simulink library "halout"  (R2021b)
settings: Solver=VariableStepAuto  StartTime=0.0  StopTime=10.0  RelTol=1e-3
undefined symbols (not defined in the file): C_TASK_5MS_S, FALSE, KHAL_CAN1FDAPS3E2E_flg, KHAL_CAN1FDAPS3TxReq_flg, KHAL_CAN1FDVCU2E2E_flg, KHAL_CAN1FDVCU2TxReq_flg, KHAL_CAN1FDVCU3E2E_flg, KHAL_CAN1FDVCU3TxReq_flg, KHAL_CAN1TxReq_flg, KHAL_CAN2TxReq_flg, KHAL_CAN3FDVCU1TxReq_flg, KHAL_CAN3FDVCU2E2E_flg, KHAL_CAN3FDVCU2TxReq_flg, KHAL_CAN3TxReq_flg, KHAL_CAN4FDVCU1E2E_flg, KHAL_CAN4FDVCU1TxReq_flg, KHAL_CAN4TxReq_flg, KHAL_CAN5TxReq_flg, ONE_INT, TRUE, ZERO_INT
libraries: FVT_lib x383, simulink x179
(part 13 of 20)

== system halout/HAL_OUT/CAN1/FD_VCU3_0x159/Byte_19 ==
  Fr_EDURealDrvOrBRgnTq : Inport
  BitwiseOR : simulink/Logic and Bit Operations/Bitwise Operator  logicop=OR  UseBitMask=off  BitMask=bin2dec('11011001')  BitMaskRealWorld=Stored Integer
  SignalPack : FVT_lib/hal/SignalPack  RightShiftCnt=0  BitMask=2^8-1  LeftShiftCnt=0
  UnitConverter : DataTypeConversion  OutDataTypeStr=uint8  RndMeth=Round
  UnitConverter1 : DataTypeConversion  OutDataTypeStr=uint16  RndMeth=Round
  convert_out : FVT_lib/hal/convert_out  gain=0.5  offset=-5300
  Byte_19 : Outport
  wires:
  BitwiseOR/1 -> Byte_19/1
  UnitConverter/1 -> BitwiseOR/1
  SignalPack/1 -> UnitConverter/1
  UnitConverter1/1 -> SignalPack/1
  convert_out/1 -> UnitConverter1/1
  Fr_EDURealDrvOrBRgnTq/1 -> convert_out/1

== system halout/HAL_OUT/CAN1/FD_VCU3_0x159/Byte_3 ==
  Fr_EDUSpdValid : Inport
  Fr_RgnDecrSta : Inport  Port=2
  Fr_RgnPermSta : Inport  Port=3
  RgnAbnorSta : Inport  Port=4
  Rr_EDUSpdValid : Inport  Port=5
  Rr_RgnDecrSta : Inport  Port=6
  Rr_RgnPermSta : Inport  Port=7
  BitwiseOR : simulink/Logic and Bit Operations/Bitwise Operator  logicop=OR  UseBitMask=off  NumInputPorts=7  BitMask=bin2dec('11011001')  BitMaskRealWorld=Stored Integer
  SignalPack : FVT_lib/hal/SignalPack  RightShiftCnt=0  BitMask=2^1-1  LeftShiftCnt=6
  SignalPack1 : FVT_lib/hal/SignalPack  RightShiftCnt=0  BitMask=2^1-1  LeftShiftCnt=3
  SignalPack2 : FVT_lib/hal/SignalPack  RightShiftCnt=0  BitMask=2^1-1  LeftShiftCnt=1
  SignalPack3 : FVT_lib/hal/SignalPack  RightShiftCnt=0  BitMask=2^1-1  LeftShiftCnt=4
  SignalPack4 : FVT_lib/hal/SignalPack  RightShiftCnt=0  BitMask=2^1-1  LeftShiftCnt=5
  SignalPack5 : FVT_lib/hal/SignalPack  RightShiftCnt=0  BitMask=2^1-1  LeftShiftCnt=2
  SignalPack6 : FVT_lib/hal/SignalPack  RightShiftCnt=0  BitMask=2^1-1  LeftShiftCnt=0
  UnitConverter{,1..13} (14 alike) : DataTypeConversion  OutDataTypeStr=uint8  RndMeth=Round
  Byte_3 : Outport
  wires:
  BitwiseOR/1 -> Byte_3/1
  UnitConverter/1 -> BitwiseOR/1
  SignalPack/1 -> UnitConverter/1
  UnitConverter1/1 -> SignalPack/1
  Fr_EDUSpdValid/1 -> UnitConverter1/1
  UnitConverter2/1 -> BitwiseOR/2
  SignalPack1/1 -> UnitConverter2/1
  UnitConverter3/1 -> SignalPack1/1
  Fr_RgnDecrSta/1 -> UnitConverter3/1
  UnitConverter4/1 -> BitwiseOR/3
  SignalPack2/1 -> UnitConverter4/1
  UnitConverter5/1 -> SignalPack2/1
  Fr_RgnPermSta/1 -> UnitConverter5/1
  UnitConverter6/1 -> BitwiseOR/4
  SignalPack3/1 -> UnitConverter6/1
  UnitConverter7/1 -> SignalPack3/1
  RgnAbnorSta/1 -> UnitConverter7/1
  UnitConverter8/1 -> BitwiseOR/5
  SignalPack4/1 -> UnitConverter8/1
  UnitConverter9/1 -> SignalPack4/1
  Rr_EDUSpdValid/1 -> UnitConverter9/1
  UnitConverter10/1 -> BitwiseOR/6
  SignalPack5/1 -> UnitConverter10/1
  UnitConverter11/1 -> SignalPack5/1
  Rr_RgnDecrSta/1 -> UnitConverter11/1
  UnitConverter12/1 -> BitwiseOR/7
  SignalPack6/1 -> UnitConverter12/1
  UnitConverter13/1 -> SignalPack6/1
  Rr_RgnPermSta/1 -> UnitConverter13/1

== system halout/HAL_OUT/CAN1/FD_VCU3_0x159/Byte_4 ==
  EquivAccPedalSWSta : Inport
  PTCS_PermSta : Inport  Port=2
  Rr_EDUSpd : Inport  Port=3
  BitwiseOR : simulink/Logic and Bit Operations/Bitwise Operator  logicop=OR  UseBitMask=off  NumInputPorts=3  BitMask=bin2dec('11011001')  BitMaskRealWorld=Stored Integer
  SignalPack : FVT_lib/hal/SignalPack  RightShiftCnt=0  BitMask=2^1-1  LeftShiftCnt=6
  SignalPack1 : FVT_lib/hal/SignalPack  RightShiftCnt=0  BitMask=2^1-1  LeftShiftCnt=7
  SignalPack2 : FVT_lib/hal/SignalPack  RightShiftCnt=8  BitMask=2^4-1  LeftShiftCnt=0
  UnitConverter{,1..4} (5 alike) : DataTypeConversion  OutDataTypeStr=uint8  RndMeth=Round
  UnitConverter5 : DataTypeConversion  OutDataTypeStr=uint16  RndMeth=Round
  convert_out : FVT_lib/hal/convert_out  gain=1  offset=-2000
  Byte_4 : Outport
  wires:
  BitwiseOR/1 -> Byte_4/1
  UnitConverter/1 -> BitwiseOR/1
  SignalPack/1 -> UnitConverter/1
  UnitConverter1/1 -> SignalPack/1
  EquivAccPedalSWSta/1 -> UnitConverter1/1
  UnitConverter2/1 -> BitwiseOR/2
  SignalPack1/1 -> UnitConverter2/1
  UnitConverter3/1 -> SignalPack1/1
  PTCS_PermSta/1 -> UnitConverter3/1
  UnitConverter4/1 -> BitwiseOR/3
  SignalPack2/1 -> UnitConverter4/1
  UnitConverter5/1 -> SignalPack2/1
  convert_out/1 -> UnitConverter5/1
  Rr_EDUSpd/1 -> convert_out/1

== system halout/HAL_OUT/CAN1/FD_VCU3_0x159/Byte_5 ==
  Rr_EDUSpd : Inport
  BitwiseOR : simulink/Logic and Bit Operations/Bitwise Operator  logicop=OR  UseBitMask=off  BitMask=bin2dec('11011001')  BitMaskRealWorld=Stored Integer
  SignalPack : FVT_lib/hal/SignalPack  RightShiftCnt=0  BitMask=2^8-1  LeftShiftCnt=0
  UnitConverter : DataTypeConversion  OutDataTypeStr=uint8  RndMeth=Round
  UnitConverter1 : DataTypeConversion  OutDataTypeStr=uint16  RndMeth=Round
  convert_out : FVT_lib/hal/convert_out  gain=1  offset=-2000
  Byte_5 : Outport
  wires:
  BitwiseOR/1 -> Byte_5/1
  UnitConverter/1 -> BitwiseOR/1
  SignalPack/1 -> UnitConverter/1
  UnitConverter1/1 -> SignalPack/1
  convert_out/1 -> UnitConverter1/1
  Rr_EDUSpd/1 -> convert_out/1

== system halout/HAL_OUT/CAN1/FD_VCU3_0x159/Byte_6 ==
  Rr_EDURealARgnTq : Inport
  BitwiseOR : simulink/Logic and Bit Operations/Bitwise Operator  logicop=OR  UseBitMask=off  BitMask=bin2dec('11011001')  BitMaskRealWorld=Stored Integer
  SignalPack : FVT_lib/hal/SignalPack  RightShiftCnt=8  BitMask=2^8-1  LeftShiftCnt=0
  UnitConverter : DataTypeConversion  OutDataTypeStr=uint8  RndMeth=Round
  UnitConverter1 : DataTypeConversion  OutDataTypeStr=uint16  RndMeth=Round
  convert_out : FVT_lib/hal/convert_out  gain=1  offset=-5300
  Byte_6 : Outport
  wires:
  BitwiseOR/1 -> Byte_6/1
  UnitConverter/1 -> BitwiseOR/1
  SignalPack/1 -> UnitConverter/1
  UnitConverter1/1 -> SignalPack/1
  convert_out/1 -> UnitConverter1/1
  Rr_EDURealARgnTq/1 -> convert_out/1

== system halout/HAL_OUT/CAN1/FD_VCU3_0x159/Byte_7 ==
  Rr_EDURealARgnTq : Inport
  BitwiseOR : simulink/Logic and Bit Operations/Bitwise Operator  logicop=OR  UseBitMask=off  BitMask=bin2dec('11011001')  BitMaskRealWorld=Stored Integer
  SignalPack : FVT_lib/hal/SignalPack  RightShiftCnt=0  BitMask=2^8-1  LeftShiftCnt=0
  UnitConverter : DataTypeConversion  OutDataTypeStr=uint8  RndMeth=Round
  UnitConverter1 : DataTypeConversion  OutDataTypeStr=uint16  RndMeth=Round
  convert_out : FVT_lib/hal/convert_out  gain=1  offset=-5300
  Byte_7 : Outport
  wires:
  BitwiseOR/1 -> Byte_7/1
  UnitConverter/1 -> BitwiseOR/1
  SignalPack/1 -> UnitConverter/1
  UnitConverter1/1 -> SignalPack/1
  convert_out/1 -> UnitConverter1/1
  Rr_EDURealARgnTq/1 -> convert_out/1

== system halout/HAL_OUT/CAN1/FD_VCU3_0x159/Byte_8 ==
  Rr_EDUAvailBrkRgnTq : Inport
  BitwiseOR : simulink/Logic and Bit Operations/Bitwise Operator  logicop=OR  UseBitMask=off  BitMask=bin2dec('11011001')  BitMaskRealWorld=Stored Integer
  SignalPack : FVT_lib/hal/SignalPack  RightShiftCnt=8  BitMask=2^8-1  LeftShiftCnt=0
  UnitConverter : DataTypeConversion  OutDataTypeStr=uint8  RndMeth=Round
  UnitConverter1 : DataTypeConversion  OutDataTypeStr=uint16  RndMeth=Round
  convert_out : FVT_lib/hal/convert_out  gain=0.5  offset=-5300
  Byte_8 : Outport
  wires:
  BitwiseOR/1 -> Byte_8/1
  UnitConverter/1 -> BitwiseOR/1
  SignalPack/1 -> UnitConverter/1
  UnitConverter1/1 -> SignalPack/1
  convert_out/1 -> UnitConverter1/1
  Rr_EDUAvailBrkRgnTq/1 -> convert_out/1

== system halout/HAL_OUT/CAN1/FD_VCU3_0x159/Byte_9 ==
  Rr_EDUAvailBrkRgnTq : Inport
  BitwiseOR : simulink/Logic and Bit Operations/Bitwise Operator  logicop=OR  UseBitMask=off  BitMask=bin2dec('11011001')  BitMaskRealWorld=Stored Integer
  SignalPack : FVT_lib/hal/SignalPack  RightShiftCnt=0  BitMask=2^8-1  LeftShiftCnt=0
  UnitConverter : DataTypeConversion  OutDataTypeStr=uint8  RndMeth=Round
  UnitConverter1 : DataTypeConversion  OutDataTypeStr=uint16  RndMeth=Round
  convert_out : FVT_lib/hal/convert_out  gain=0.5  offset=-5300
  Byte_9 : Outport
  wires:
  BitwiseOR/1 -> Byte_9/1
  UnitConverter/1 -> BitwiseOR/1
  SignalPack/1 -> UnitConverter/1
  UnitConverter1/1 -> SignalPack/1
  convert_out/1 -> UnitConverter1/1
  Rr_EDUAvailBrkRgnTq/1 -> convert_out/1

== system halout/HAL_OUT/CAN1/FD_VCU3_0x159/CSVCU3CAN1 ==
  CSVCU3CAN1 : Inport
  Data Type Conversion : DataTypeConversion  OutDataTypeStr=uint8  RndMeth=Round
  CAN1_CS_VCU3_CAN1 : Outport
  wires:
  Data Type Conversion/1 -> CAN1_CS_VCU3_CAN1/1
  CSVCU3CAN1/1 -> Data Type Conversion/1

== system halout/HAL_OUT/CAN1/FD_VCU3_0x159/EquivAccPedalSWSta ==
  EquivAccPedalSWSta : Inport
  Data Type Conversion : DataTypeConversion  OutDataTypeStr=uint8  RndMeth=Round
  CAN1_EquivAccPedalSWSta : Outport
  wires:
  Data Type Conversion/1 -> CAN1_EquivAccPedalSWSta/1
  EquivAccPedalSWSta/1 -> Data Type Conversion/1

== system halout/HAL_OUT/CAN1/FD_VCU3_0x159/FrEDUAvailBrkRgnTq ==
  FrEDUAvailBrkRgnTq : Inport
  Data Type Conversion : DataTypeConversion  OutDataTypeStr=uint16  RndMeth=Round
  convert_out : FVT_lib/hal/convert_out  gain=0.5  offset=-5300
  CAN1_Fr_EDUAvailBrkRgnTq : Outport
  wires:
  Data Type Conversion/1 -> CAN1_Fr_EDUAvailBrkRgnTq/1
  convert_out/1 -> Data Type Conversion/1
  FrEDUAvailBrkRgnTq/1 -> convert_out/1

== system halout/HAL_OUT/CAN1/FD_VCU3_0x159/FrEDUAvailBrkRgnTqValid ==
  FrEDUAvailBrkRgnTqValid : Inport
  Data Type Conversion : DataTypeConversion  OutDataTypeStr=uint8  RndMeth=Round
  CAN1_Fr_EDUAvailBrkRgnTqValid : Outport
  wires:
  Data Type Conversion/1 -> CAN1_Fr_EDUAvailBrkRgnTqValid/1
  FrEDUAvailBrkRgnTqValid/1 -> Data Type Conversion/1

== system halout/HAL_OUT/CAN1/FD_VCU3_0x159/FrEDURealARgnTq ==
  FrEDURealARgnTq : Inport
  Data Type Conversion : DataTypeConversion  OutDataTypeStr=uint16  RndMeth=Round
  convert_out : FVT_lib/hal/convert_out  gain=1  offset=-5300
  CAN1_Fr_EDURealARgnTq : Outport
  wires:
  Data Type Conversion/1 -> CAN1_Fr_EDURealARgnTq/1
  convert_out/1 -> Data Type Conversion/1
  FrEDURealARgnTq/1 -> convert_out/1

== system halout/HAL_OUT/CAN1/FD_VCU3_0x159/FrEDURealDrvOrBRgnTq ==
  FrEDURealDrvOrBRgnTq : Inport
  Data Type Conversion : DataTypeConversion  OutDataTypeStr=uint16  RndMeth=Round
  convert_out : FVT_lib/hal/convert_out  gain=0.5  offset=-5300
  CAN1_Fr_EDURealDrvOrBRgnTq : Outport
  wires:
  Data Type Conversion/1 -> CAN1_Fr_EDURealDrvOrBRgnTq/1
  convert_out/1 -> Data Type Conversion/1
  FrEDURealDrvOrBRgnTq/1 -> convert_out/1

== system halout/HAL_OUT/CAN1/FD_VCU3_0x159/FrEDUSpd ==
  FrEDUSpd : Inport
  Data Type Conversion : DataTypeConversion  OutDataTypeStr=uint16  RndMeth=Round
  convert_out : FVT_lib/hal/convert_out  gain=1  offset=-2000
  CAN1_Fr_EDUSpd : Outport
  wires:
  Data Type Conversion/1 -> CAN1_Fr_EDUSpd/1
  convert_out/1 -> Data Type Conversion/1
  FrEDUSpd/1 -> convert_out/1

== system halout/HAL_OUT/CAN1/FD_VCU3_0x159/FrEDUSpdValid ==
  FrEDUSpdValid : Inport
  Data Type Conversion : DataTypeConversion  OutDataTypeStr=uint8  RndMeth=Round
  CAN1_Fr_EDUSpdValid : Outport
  wires:
  Data Type Conversion/1 -> CAN1_Fr_EDUSpdValid/1
  FrEDUSpdValid/1 -> Data Type Conversion/1

== system halout/HAL_OUT/CAN1/FD_VCU3_0x159/FrRgnDecrSta ==
  FrRgnDecrSta : Inport
  Data Type Conversion : DataTypeConversion  OutDataTypeStr=uint8  RndMeth=Round
  CAN1_Fr_RgnDecrSta : Outport
  wires:
  Data Type Conversion/1 -> CAN1_Fr_RgnDecrSta/1
  FrRgnDecrSta/1 -> Data Type Conversion/1

== system halout/HAL_OUT/CAN1/FD_VCU3_0x159/FrRgnPermSta ==
  FrRgnPermSta : Inport
  Data Type Conversion : DataTypeConversion  OutDataTypeStr=uint8  RndMeth=Round
  CAN1_Fr_RgnPermSta : Outport
  wires:
  Data Type Conversion/1 -> CAN1_Fr_RgnPermSta/1
  FrRgnPermSta/1 -> Data Type Conversion/1

== system halout/HAL_OUT/CAN1/FD_VCU3_0x159/PTCSPermSta ==
  PTCSPermSta : Inport
  Data Type Conversion : DataTypeConversion  OutDataTypeStr=uint8  RndMeth=Round
  CAN1_PTCS_PermSta : Outport
  wires:
  Data Type Conversion/1 -> CAN1_PTCS_PermSta/1
  PTCSPermSta/1 -> Data Type Conversion/1

== system halout/HAL_OUT/CAN1/FD_VCU3_0x159/RCVCU3CAN1 ==
  RCVCU3CAN1 : Inport
  Data Type Conversion : DataTypeConversion  OutDataTypeStr=uint8  RndMeth=Round
  CAN1_RC_VCU3_CAN1 : Outport
  wires:
  Data Type Conversion/1 -> CAN1_RC_VCU3_CAN1/1
  RCVCU3CAN1/1 -> Data Type Conversion/1

== system halout/HAL_OUT/CAN1/FD_VCU3_0x159/RgnAbnorSta ==
  RgnAbnorSta : Inport
  Data Type Conversion : DataTypeConversion  OutDataTypeStr=uint8  RndMeth=Round
  CAN1_RgnAbnorSta : Outport
  wires:
  Data Type Conversion/1 -> CAN1_RgnAbnorSta/1
  RgnAbnorSta/1 -> Data Type Conversion/1

== system halout/HAL_OUT/CAN1/FD_VCU3_0x159/RrEDUAvailBrkRgnTq ==
  RrEDUAvailBrkRgnTq : Inport
  Data Type Conversion : DataTypeConversion  OutDataTypeStr=uint16  RndMeth=Round
  convert_out : FVT_lib/hal/convert_out  gain=0.5  offset=-5300
  CAN1_Rr_EDUAvailBrkRgnTq : Outport
  wires:
  Data Type Conversion/1 -> CAN1_Rr_EDUAvailBrkRgnTq/1
  convert_out/1 -> Data Type Conversion/1
  RrEDUAvailBrkRgnTq/1 -> convert_out/1

== system halout/HAL_OUT/CAN1/FD_VCU3_0x159/RrEDUAvailBrkRgnTqValid ==
  RrEDUAvailBrkRgnTqValid : Inport
  Data Type Conversion : DataTypeConversion  OutDataTypeStr=uint8  RndMeth=Round
  CAN1_Rr_EDUAvailBrkRgnTqValid : Outport
  wires:
  Data Type Conversion/1 -> CAN1_Rr_EDUAvailBrkRgnTqValid/1
  RrEDUAvailBrkRgnTqValid/1 -> Data Type Conversion/1

== system halout/HAL_OUT/CAN1/FD_VCU3_0x159/RrEDURealARgnTq ==
  RrEDURealARgnTq : Inport
  Data Type Conversion : DataTypeConversion  OutDataTypeStr=uint16  RndMeth=Round
  convert_out : FVT_lib/hal/convert_out  gain=1  offset=-5300
  CAN1_Rr_EDURealARgnTq : Outport
  wires:
  Data Type Conversion/1 -> CAN1_Rr_EDURealARgnTq/1
  convert_out/1 -> Data Type Conversion/1
  RrEDURealARgnTq/1 -> convert_out/1

== system halout/HAL_OUT/CAN1/FD_VCU3_0x159/RrEDURealDrvOrBRgnTq ==
  RrEDURealDrvOrBRgnTq : Inport
  Data Type Conversion : DataTypeConversion  OutDataTypeStr=uint16  RndMeth=Round
  convert_out : FVT_lib/hal/convert_out  gain=0.5  offset=-5300
  CAN1_Rr_EDURealDrvOrBRgnTq : Outport
  wires:
  Data Type Conversion/1 -> CAN1_Rr_EDURealDrvOrBRgnTq/1
  convert_out/1 -> Data Type Conversion/1
  RrEDURealDrvOrBRgnTq/1 -> convert_out/1

== system halout/HAL_OUT/CAN1/FD_VCU3_0x159/RrEDUSpd ==
  RrEDUSpd : Inport
  Data Type Conversion : DataTypeConversion  OutDataTypeStr=uint16  RndMeth=Round
  convert_out : FVT_lib/hal/convert_out  gain=1  offset=-2000
  CAN1_Rr_EDUSpd : Outport
  wires:
  Data Type Conversion/1 -> CAN1_Rr_EDUSpd/1
  convert_out/1 -> Data Type Conversion/1
  RrEDUSpd/1 -> convert_out/1

== system halout/HAL_OUT/CAN1/FD_VCU3_0x159/RrEDUSpdValid ==
  RrEDUSpdValid : Inport
  Data Type Conversion : DataTypeConversion  OutDataTypeStr=uint8  RndMeth=Round
  CAN1_Rr_EDUSpdValid : Outport
  wires:
  Data Type Conversion/1 -> CAN1_Rr_EDUSpdValid/1
  RrEDUSpdValid/1 -> Data Type Conversion/1

== system halout/HAL_OUT/CAN1/FD_VCU3_0x159/RrRgnDecrSta ==
  RrRgnDecrSta : Inport
  Data Type Conversion : DataTypeConversion  OutDataTypeStr=uint8  RndMeth=Round
  CAN1_Rr_RgnDecrSta : Outport
  wires:
  Data Type Conversion/1 -> CAN1_Rr_RgnDecrSta/1
  RrRgnDecrSta/1 -> Data Type Conversion/1

== system halout/HAL_OUT/CAN1/FD_VCU3_0x159/RrRgnPermSta ==
  RrRgnPermSta : Inport
  Data Type Conversion : DataTypeConversion  OutDataTypeStr=uint8  RndMeth=Round
  CAN1_Rr_RgnPermSta : Outport
  wires:
  Data Type Conversion/1 -> CAN1_Rr_RgnPermSta/1
  RrRgnPermSta/1 -> Data Type Conversion/1

== system halout/HAL_OUT/CAN1/FD_VCU4_0x3C0/EngAGSCloseSta ==
  EngAGSCloseSta : Inport
  Data Type Conversion : DataTypeConversion  OutDataTypeStr=uint8  RndMeth=Round
  CAN1_Eng_AGSCloseSta : Outport
  wires:
  Data Type Conversion/1 -> CAN1_Eng_AGSCloseSta/1
  EngAGSCloseSta/1 -> Data Type Conversion/1

== system halout/HAL_OUT/CAN1/FD_VCU4_0x3C0/EngActvDmpDisabSta ==
  EngActvDmpDisabSta : Inport
  Data Type Conversion : DataTypeConversion  OutDataTypeStr=uint8  RndMeth=Round
  CAN1_Eng_ActvDmpDisabSta : Outport
  wires:
  Data Type Conversion/1 -> CAN1_Eng_ActvDmpDisabSta/1
  EngActvDmpDisabSta/1 -> Data Type Conversion/1

== system halout/HAL_OUT/CAN1/FD_VCU4_0x3C0/EngCoastDwSta ==
  EngCoastDwSta : Inport
  Data Type Conversion : DataTypeConversion  OutDataTypeStr=uint8  RndMeth=Round
  CAN1_Eng_CoastDwSta : Outport
  wires:
  Data Type Conversion/1 -> CAN1_Eng_CoastDwSta/1
  EngCoastDwSta/1 -> Data Type Conversion/1

== system halout/HAL_OUT/CAN1/FD_VCU4_0x3C0/EngPwrLockSta ==
  EngPwrLockSta : Inport
  Data Type Conversion : DataTypeConversion  OutDataTypeStr=uint8  RndMeth=Round
  CAN1_Eng_PwrLockSta : Outport
  wires:
  Data Type Conversion/1 -> CAN1_Eng_PwrLockSta/1
  EngPwrLockSta/1 -> Data Type Conversion/1

== system halout/HAL_OUT/CAN1/FD_VCU4_0x3C0/VehMalfunLevel ==
  VehMalfunLevel : Inport
  Data Type Conversion : DataTypeConversion  OutDataTypeStr=uint8  RndMeth=Round
  CAN1_VehMalfunLevel : Outport
  wires:
  Data Type Conversion/1 -> CAN1_VehMalfunLevel/1
  VehMalfunLevel/1 -> Data Type Conversion/1

== system halout/HAL_OUT/CAN2/FD_APS1_0x236/APSAngleTarget ==
  APSAngleTarget : Inport
  Data Type Conversion : DataTypeConversion  OutDataTypeStr=uint16  RndMeth=Round
  convert_out : FVT_lib/hal/convert_out  gain=0.1  offset=-900
  CAN2_APS_Angle_Target : Outport
  wires:
  Data Type Conversion/1 -> CAN2_APS_Angle_Target/1
  convert_out/1 -> Data Type Conversion/1
  APSAngleTarget/1 -> convert_out/1

== system halout/HAL_OUT/CAN2/FD_APS1_0x236/APSRqEPASCtrl ==
  APSRqEPASCtrl : Inport
  Data Type Conversion : DataTypeConversion  OutDataTypeStr=uint8  RndMeth=Round
  CAN2_APS_Rq_EPAS_Ctrl : Outport
  wires:
  Data Type Conversion/1 -> CAN2_APS_Rq_EPAS_Ctrl/1
  APSRqEPASCtrl/1 -> Data Type Conversion/1

== system halout/HAL_OUT/CAN2/FD_APS1_0x236/APSStaSystem ==
  APSStaSystem : Inport
  Data Type Conversion : DataTypeConversion  OutDataTypeStr=uint8  RndMeth=Round
  CAN2_APS_Sta_System : Outport
  wires:
  Data Type Conversion/1 -> CAN2_APS_Sta_System/1
  APSStaSystem/1 -> Data Type Conversion/1

== system halout/HAL_OUT/CAN2/FD_APS1_0x236/APSVRqEPASCtrl ==
  APSVRqEPASCtrl : Inport
  Data Type Conversion : DataTypeConversion  OutDataTypeStr=uint8  RndMeth=Round
  CAN2_APS_V_Rq_EPAS_Ctrl : Outport
  wires:
  Data Type Conversion/1 -> CAN2_APS_V_Rq_EPAS_Ctrl/1
  APSVRqEPASCtrl/1 -> Data Type Conversion/1

== system halout/HAL_OUT/CAN2/FD_APS2_0x210/APSDFLL ==
  APSDFLL : Inport
  Data Type Conversion : DataTypeConversion  OutDataTypeStr=uint16  RndMeth=Round
  CAN2_APS_D_FLL : Outport
  wires:
  Data Type Conversion/1 -> CAN2_APS_D_FLL/1
  APSDFLL/1 -> Data Type Conversion/1

== system halout/HAL_OUT/CAN2/FD_APS2_0x210/APSDFLR ==
  APSDFLR : Inport
  Data Type Conversion : DataTypeConversion  OutDataTypeStr=uint16  RndMeth=Round
  CAN2_APS_D_FLR : Outport
  wires:
  Data Type Conversion/1 -> CAN2_APS_D_FLR/1
  APSDFLR/1 -> Data Type Conversion/1

== system halout/HAL_OUT/CAN2/FD_APS2_0x210/APSDRLL ==
  APSDRLL : Inport
  Data Type Conversion : DataTypeConversion  OutDataTypeStr=uint16  RndMeth=Round
  CAN2_APS_D_RLL : Outport
  wires:
  Data Type Conversion/1 -> CAN2_APS_D_RLL/1
  APSDRLL/1 -> Data Type Conversion/1

== system halout/HAL_OUT/CAN2/FD_APS2_0x210/APSDRLR ==
  APSDRLR : Inport
  Data Type Conversion : DataTypeConversion  OutDataTypeStr=uint16  RndMeth=Round
  CAN2_APS_D_RLR : Outport
  wires:
  Data Type Conversion/1 -> CAN2_APS_D_RLR/1
  APSDRLR/1 -> Data Type Conversion/1

== system halout/HAL_OUT/CAN2/FD_APS2_0x210/APSExitCondition ==
  APSExitCondition : Inport
  Data Type Conversion : DataTypeConversion  OutDataTypeStr=uint8  RndMeth=Round
  CAN2_APS_ExitCondition : Outport
  wires:
  Data Type Conversion/1 -> CAN2_APS_ExitCondition/1
  APSExitCondition/1 -> Data Type Conversion/1

== system halout/HAL_OUT/CAN2/FD_APS2_0x210/APSHWVer ==
  APSHWVer : Inport
  Data Type Conversion : DataTypeConversion  OutDataTypeStr=uint8  RndMeth=Round
  CAN2_APS_HW_Ver : Outport
  wires:
  Data Type Conversion/1 -> CAN2_APS_HW_Ver/1
  APSHWVer/1 -> Data Type Conversion/1

== system halout/HAL_OUT/CAN2/FD_APS2_0x210/APSProgressPCT ==
  APSProgressPCT : Inport
  Data Type Conversion : DataTypeConversion  OutDataTypeStr=uint8  RndMeth=Round
  CAN2_APS_Progress_PCT : Outport
  wires:
  Data Type Conversion/1 -> CAN2_APS_Progress_PCT/1
  APSProgressPCT/1 -> Data Type Conversion/1

== system halout/HAL_OUT/CAN2/FD_APS2_0x210/APSRQDisplay ==
  APSRQDisplay : Inport
  Data Type Conversion : DataTypeConversion  OutDataTypeStr=uint8  RndMeth=Round
  CAN2_APS_RQ_Display : Outport
  wires:
  Data Type Conversion/1 -> CAN2_APS_RQ_Display/1
  APSRQDisplay/1 -> Data Type Conversion/1

== system halout/HAL_OUT/CAN2/FD_APS2_0x210/APSSWVer ==
  APSSWVer : Inport
  Data Type Conversion : DataTypeConversion  OutDataTypeStr=uint8  RndMeth=Round
  CAN2_APS_SW_Ver : Outport
  wires:
  Data Type Conversion/1 -> CAN2_APS_SW_Ver/1
  APSSWVer/1 -> Data Type Conversion/1

== system halout/HAL_OUT/CAN2/FD_APS2_0x210/FDCVCURegenLimIndSta ==
  FDCVCURegenLimIndSta : Inport
  Data Type Conversion : DataTypeConversion  OutDataTypeStr=uint8  RndMeth=Round
  CAN2_FDC_VCU_RegenLimInd_Sta : Outport
  wires:
  Data Type Conversion/1 -> CAN2_FDC_VCU_RegenLimInd_Sta/1
  FDCVCURegenLimIndSta/1 -> Data Type Conversion/1

== system halout/HAL_OUT/CAN2/FD_APS2_0x210/FDCVCUSmartEcoSpdLimSta ==
  FDCVCUSmartEcoSpdLimSta : Inport
  Data Type Conversion : DataTypeConversion  OutDataTypeStr=uint8  RndMeth=Round
  CAN2_FDC_VCU_SmartEcoSpdLim_Sta : Outport
  wires:
  Data Type Conversion/1 -> CAN2_FDC_VCU_SmartEcoSpdLim_Sta/1
  FDCVCUSmartEcoSpdLimSta/1 -> Data Type Conversion/1

== system halout/HAL_OUT/CAN2/FD_APS2_0x210/FDCVCUSmartEcoSta ==
  FDCVCUSmartEcoSta : Inport
  Data Type Conversion : DataTypeConversion  OutDataTypeStr=uint8  RndMeth=Round
  CAN2_FDC_VCU_SmartEco_Sta : Outport
  wires:
  Data Type Conversion/1 -> CAN2_FDC_VCU_SmartEco_Sta/1
  FDCVCUSmartEcoSta/1 -> Data Type Conversion/1

== system halout/HAL_OUT/CAN2/FD_APS2_0x210/PASAFCL ==
  PASAFCL : Inport
  Data Type Conversion : DataTypeConversion  OutDataTypeStr=uint8  RndMeth=Round
  CAN2_PAS_A_FCL : Outport
  wires:
  Data Type Conversion/1 -> CAN2_PAS_A_FCL/1
  PASAFCL/1 -> Data Type Conversion/1

== system halout/HAL_OUT/CAN2/FD_APS2_0x210/PASAFCR ==
  PASAFCR : Inport
  Data Type Conversion : DataTypeConversion  OutDataTypeStr=uint8  RndMeth=Round
  CAN2_PAS_A_FCR : Outport
  wires:
  Data Type Conversion/1 -> CAN2_PAS_A_FCR/1
  PASAFCR/1 -> Data Type Conversion/1

== system halout/HAL_OUT/CAN2/FD_APS2_0x210/PASAFML ==
  PASAFML : Inport
  Data Type Conversion : DataTypeConversion  OutDataTypeStr=uint8  RndMeth=Round
  CAN2_PAS_A_FML : Outport
  wires:
  Data Type Conversion/1 -> CAN2_PAS_A_FML/1
  PASAFML/1 -> Data Type Conversion/1

== system halout/HAL_OUT/CAN2/FD_APS2_0x210/PASAFMR ==
  PASAFMR : Inport
  Data Type Conversion : DataTypeConversion  OutDataTypeStr=uint8  RndMeth=Round
  CAN2_PAS_A_FMR : Outport
  wires:
  Data Type Conversion/1 -> CAN2_PAS_A_FMR/1
  PASAFMR/1 -> Data Type Conversion/1

== system halout/HAL_OUT/CAN2/FD_APS2_0x210/PASARCL ==
  PASARCL : Inport
  Data Type Conversion : DataTypeConversion  OutDataTypeStr=uint8  RndMeth=Round
  CAN2_PAS_A_RCL : Outport
  wires:
  Data Type Conversion/1 -> CAN2_PAS_A_RCL/1
  PASARCL/1 -> Data Type Conversion/1

== system halout/HAL_OUT/CAN2/FD_APS2_0x210/PASARCR ==
  PASARCR : Inport
  Data Type Conversion : DataTypeConversion  OutDataTypeStr=uint8  RndMeth=Round
  CAN2_PAS_A_RCR : Outport
  wires:
  Data Type Conversion/1 -> CAN2_PAS_A_RCR/1
  PASARCR/1 -> Data Type Conversion/1

== system halout/HAL_OUT/CAN2/FD_APS2_0x210/PASARML ==
  PASARML : Inport
  Data Type Conversion : DataTypeConversion  OutDataTypeStr=uint8  RndMeth=Round
  CAN2_PAS_A_RML : Outport
  wires:
  Data Type Conversion/1 -> CAN2_PAS_A_RML/1
  PASARML/1 -> Data Type Conversion/1

== system halout/HAL_OUT/CAN2/FD_APS2_0x210/PASARMR ==
  PASARMR : Inport
  Data Type Conversion : DataTypeConversion  OutDataTypeStr=uint8  RndMeth=Round
  CAN2_PAS_A_RMR : Outport
  wires:
  Data Type Conversion/1 -> CAN2_PAS_A_RMR/1
  PASARMR/1 -> Data Type Conversion/1

== system halout/HAL_OUT/CAN2/FD_APS2_0x210/PASChime ==
  PASChime : Inport
  Data Type Conversion : DataTypeConversion  OutDataTypeStr=uint8  RndMeth=Round
  CAN2_PAS_Chime : Outport
  wires:
  Data Type Conversion/1 -> CAN2_PAS_Chime/1
  PASChime/1 -> Data Type Conversion/1

== system halout/HAL_OUT/CAN2/FD_APS2_0x210/PASDFCL ==
  PASDFCL : Inport
  Data Type Conversion : DataTypeConversion  OutDataTypeStr=uint8  RndMeth=Round
  CAN2_PAS_D_FCL : Outport
  wires:
  Data Type Conversion/1 -> CAN2_PAS_D_FCL/1
  PASDFCL/1 -> Data Type Conversion/1

== system halout/HAL_OUT/CAN2/FD_APS2_0x210/PASDFCR ==
  PASDFCR : Inport
  Data Type Conversion : DataTypeConversion  OutDataTypeStr=uint8  RndMeth=Round
  CAN2_PAS_D_FCR : Outport
  wires:
  Data Type Conversion/1 -> CAN2_PAS_D_FCR/1
  PASDFCR/1 -> Data Type Conversion/1

== system halout/HAL_OUT/CAN2/FD_APS2_0x210/PASDFML ==
  PASDFML : Inport
  Data Type Conversion : DataTypeConversion  OutDataTypeStr=uint8  RndMeth=Round
  CAN2_PAS_D_FML : Outport
  wires:
  Data Type Conversion/1 -> CAN2_PAS_D_FML/1
  PASDFML/1 -> Data Type Conversion/1

== system halout/HAL_OUT/CAN2/FD_APS2_0x210/PASDFMR ==
  PASDFMR : Inport
  Data Type Conversion : DataTypeConversion  OutDataTypeStr=uint8  RndMeth=Round
  CAN2_PAS_D_FMR : Outport
  wires:
  Data Type Conversion/1 -> CAN2_PAS_D_FMR/1
  PASDFMR/1 -> Data Type Conversion/1

== system halout/HAL_OUT/CAN2/FD_APS2_0x210/PASDRCL ==
  PASDRCL : Inport
  Data Type Conversion : DataTypeConversion  OutDataTypeStr=uint8  RndMeth=Round
  CAN2_PAS_D_RCL : Outport
  wires:
  Data Type Conversion/1 -> CAN2_PAS_D_RCL/1
  PASDRCL/1 -> Data Type Conversion/1

== system halout/HAL_OUT/CAN2/FD_APS2_0x210/PASDRCR ==
  PASDRCR : Inport
  Data Type Conversion : DataTypeConversion  OutDataTypeStr=uint8  RndMeth=Round
  CAN2_PAS_D_RCR : Outport
  wires:
  Data Type Conversion/1 -> CAN2_PAS_D_RCR/1
  PASDRCR/1 -> Data Type Conversion/1

== system halout/HAL_OUT/CAN2/FD_APS2_0x210/PASDRML ==
  PASDRML : Inport
  Data Type Conversion : DataTypeConversion  OutDataTypeStr=uint8  RndMeth=Round
  CAN2_PAS_D_RML : Outport
  wires:
  Data Type Conversion/1 -> CAN2_PAS_D_RML/1
  PASDRML/1 -> Data Type Conversion/1

== system halout/HAL_OUT/CAN2/FD_APS2_0x210/PASDRMR ==
  PASDRMR : Inport
  Data Type Conversion : DataTypeConversion  OutDataTypeStr=uint8  RndMeth=Round
  CAN2_PAS_D_RMR : Outport
  wires:
  Data Type Conversion/1 -> CAN2_PAS_D_RMR/1
  PASDRMR/1 -> Data Type Conversion/1

== system halout/HAL_OUT/CAN2/FD_APS2_0x210/PASModOperation ==
  PASModOperation : Inport
  Data Type Conversion : DataTypeConversion  OutDataTypeStr=uint8  RndMeth=Round
  CAN2_PAS_Mod_Operation : Outport
  wires:
  Data Type Conversion/1 -> CAN2_PAS_Mod_Operation/1
  PASModOperation/1 -> Data Type Conversion/1

== system halout/HAL_OUT/CAN2/FD_APS2_0x210/PASSNSRLayout ==
  PASSNSRLayout : Inport
  Data Type Conversion : DataTypeConversion  OutDataTypeStr=uint8  RndMeth=Round
  CAN2_PAS_SNSR_Layout : Outport
  wires:
  Data Type Conversion/1 -> CAN2_PAS_SNSR_Layout/1
  PASSNSRLayout/1 -> Data Type Conversion/1

== system halout/HAL_OUT/CAN2/FD_APS2_0x210/PASStaFSys ==
  PASStaFSys : Inport
  Data Type Conversion : DataTypeConversion  OutDataTypeStr=uint8  RndMeth=Round
  CAN2_PAS_Sta_F_Sys : Outport
  wires:
  Data Type Conversion/1 -> CAN2_PAS_Sta_F_Sys/1
  PASStaFSys/1 -> Data Type Conversion/1

== system halout/HAL_OUT/CAN2/FD_APS2_0x210/USSStaFCL ==
  USSStaFCL : Inport
  Data Type Conversion : DataTypeConversion  OutDataTypeStr=uint8  RndMeth=Round
  CAN2_USS_Sta_FCL : Outport
  wires:
  Data Type Conversion/1 -> CAN2_USS_Sta_FCL/1
  USSStaFCL/1 -> Data Type Conversion/1

== system halout/HAL_OUT/CAN2/FD_APS2_0x210/USSStaFCR ==
  USSStaFCR : Inport
  Data Type Conversion : DataTypeConversion  OutDataTypeStr=uint8  RndMeth=Round
  CAN2_USS_Sta_FCR : Outport
  wires:
  Data Type Conversion/1 -> CAN2_USS_Sta_FCR/1
  USSStaFCR/1 -> Data Type Conversion/1

== system halout/HAL_OUT/CAN2/FD_APS2_0x210/USSStaFLL ==
  USSStaFLL : Inport
  Data Type Conversion : DataTypeConversion  OutDataTypeStr=uint8  RndMeth=Round
  CAN2_USS_Sta_FLL : Outport
  wires:
  Data Type Conversion/1 -> CAN2_USS_Sta_FLL/1
  USSStaFLL/1 -> Data Type Conversion/1

== system halout/HAL_OUT/CAN2/FD_APS2_0x210/USSStaFLR ==
  USSStaFLR : Inport
  Data Type Conversion : DataTypeConversion  OutDataTypeStr=uint8  RndMeth=Round
  CAN2_USS_Sta_FLR : Outport
  wires:
  Data Type Conversion/1 -> CAN2_USS_Sta_FLR/1
  USSStaFLR/1 -> Data Type Conversion/1

== system halout/HAL_OUT/CAN2/FD_APS2_0x210/USSStaFML ==
  USSStaFML : Inport
  Data Type Conversion : DataTypeConversion  OutDataTypeStr=uint8  RndMeth=Round
  CAN2_USS_Sta_FML : Outport
  wires:
  Data Type Conversion/1 -> CAN2_USS_Sta_FML/1
  USSStaFML/1 -> Data Type Conversion/1

== system halout/HAL_OUT/CAN2/FD_APS2_0x210/USSStaFMR ==
  USSStaFMR : Inport
  Data Type Conversion : DataTypeConversion  OutDataTypeStr=uint8  RndMeth=Round
  CAN2_USS_Sta_FMR : Outport
  wires:
  Data Type Conversion/1 -> CAN2_USS_Sta_FMR/1
  USSStaFMR/1 -> Data Type Conversion/1

== system halout/HAL_OUT/CAN2/FD_APS2_0x210/USSStaRCL ==
  USSStaRCL : Inport
  Data Type Conversion : DataTypeConversion  OutDataTypeStr=uint8  RndMeth=Round
  CAN2_USS_Sta_RCL : Outport
  wires:
  Data Type Conversion/1 -> CAN2_USS_Sta_RCL/1
  USSStaRCL/1 -> Data Type Conversion/1

== system halout/HAL_OUT/CAN2/FD_APS2_0x210/USSStaRCR ==
  USSStaRCR : Inport
  Data Type Conversion : DataTypeConversion  OutDataTypeStr=uint8  RndMeth=Round
  CAN2_USS_Sta_RCR : Outport
  wires:
  Data Type Conversion/1 -> CAN2_USS_Sta_RCR/1
  USSStaRCR/1 -> Data Type Conversion/1

== system halout/HAL_OUT/CAN2/FD_APS2_0x210/USSStaRLL ==
  USSStaRLL : Inport
  Data Type Conversion : DataTypeConversion  OutDataTypeStr=uint8  RndMeth=Round
  CAN2_USS_Sta_RLL : Outport
  wires:
  Data Type Conversion/1 -> CAN2_USS_Sta_RLL/1
  USSStaRLL/1 -> Data Type Conversion/1

== system halout/HAL_OUT/CAN2/FD_APS2_0x210/USSStaRLR ==
  USSStaRLR : Inport
  Data Type Conversion : DataTypeConversion  OutDataTypeStr=uint8  RndMeth=Round
  CAN2_USS_Sta_RLR : Outport
  wires:
  Data Type Conversion/1 -> CAN2_USS_Sta_RLR/1
  USSStaRLR/1 -> Data Type Conversion/1

== system halout/HAL_OUT/CAN2/FD_APS2_0x210/USSStaRML ==
  USSStaRML : Inport
  Data Type Conversion : DataTypeConversion  OutDataTypeStr=uint8  RndMeth=Round
  CAN2_USS_Sta_RML : Outport
  wires:
  Data Type Conversion/1 -> CAN2_USS_Sta_RML/1
  USSStaRML/1 -> Data Type Conversion/1

== system halout/HAL_OUT/CAN2/FD_APS2_0x210/USSStaRMR ==
  USSStaRMR : Inport
  Data Type Conversion : DataTypeConversion  OutDataTypeStr=uint8  RndMeth=Round
  CAN2_USS_Sta_RMR : Outport
  wires:
  Data Type Conversion/1 -> CAN2_USS_Sta_RMR/1
  USSStaRMR/1 -> Data Type Conversion/1

== system halout/HAL_OUT/CAN2/FD_APS3_0x238/APS3LifeCount ==
  APS3LifeCount : Inport
  Data Type Conversion : DataTypeConversion  OutDataTypeStr=uint8  RndMeth=Round
  CAN2_APS3_LifeCount : Outport
  wires:
  Data Type Conversion/1 -> CAN2_APS3_LifeCount/1
  APS3LifeCount/1 -> Data Type Conversion/1

== system halout/HAL_OUT/CAN2/FD_APS3_0x238/APS3checksum ==
  APS3checksum : Inport
  Data Type Conversion : DataTypeConversion  OutDataTypeStr=uint8  RndMeth=Round
  CAN2_APS3_checksum : Outport
  wires:
  Data Type Conversion/1 -> CAN2_APS3_checksum/1
  APS3checksum/1 -> Data Type Conversion/1

== system halout/HAL_OUT/CAN2/FD_APS3_0x238/APSDecReq ==
  APSDecReq : Inport
  Data Type Conversion : DataTypeConversion  OutDataTypeStr=uint8  RndMeth=Round
  convert_out : FVT_lib/hal/convert_out  gain=0.1  offset=0
  CAN2_APS_DecReq : Outport
  wires:
  Data Type Conversion/1 -> CAN2_APS_DecReq/1
  convert_out/1 -> Data Type Conversion/1
  APSDecReq/1 -> convert_out/1

== system halout/HAL_OUT/CAN2/FD_APS3_0x238/APSDecReqA ==
  APSDecReqA : Inport
  Data Type Conversion : DataTypeConversion  OutDataTypeStr=uint8  RndMeth=Round
  CAN2_APS_DecReq_A : Outport
  wires:
  Data Type Conversion/1 -> CAN2_APS_DecReq_A/1
  APSDecReqA/1 -> Data Type Conversion/1

== system halout/HAL_OUT/CAN2/FD_APS3_0x238/APSOpenPTG ==
  APSOpenPTG : Inport
  Data Type Conversion : DataTypeConversion  OutDataTypeStr=uint8  RndMeth=Round
  CAN2_APSOpenPTG : Outport
  wires:
  Data Type Conversion/1 -> CAN2_APSOpenPTG/1
  APSOpenPTG/1 -> Data Type Conversion/1

== system halout/HAL_OUT/CAN2/FD_APS3_0x238/APSReq ==
  APSReq : Inport
  Data Type Conversion : DataTypeConversion  OutDataTypeStr=uint8  RndMeth=Round
  CAN2_APS_Req : Outport
  wires:
  Data Type Conversion/1 -> CAN2_APS_Req/1
  APSReq/1 -> Data Type Conversion/1

== system halout/HAL_OUT/CAN2/FD_APS3_0x238/CAASSta ==
  CAASSta : Inport
  Data Type Conversion : DataTypeConversion  OutDataTypeStr=uint8  RndMeth=Round
  CAN2_CAAS_Sta : Outport
  wires:
  Data Type Conversion/1 -> CAN2_CAAS_Sta/1
  CAASSta/1 -> Data Type Conversion/1

== system halout/HAL_OUT/CAN2/FD_APS3_0x238/SPTGDet ==
  SPTGDet : Inport
  Data Type Conversion : DataTypeConversion  OutDataTypeStr=uint8  RndMeth=Round
  CAN2_SPTGDet : Outport
  wires:
  Data Type Conversion/1 -> CAN2_SPTGDet/1
  SPTGDet/1 -> Data Type Conversion/1

== system halout/HAL_OUT/CAN2/FD_APS3_0x238/SPTGSta ==
  SPTGSta : Inport
  Data Type Conversion : DataTypeConversion  OutDataTypeStr=uint8  RndMeth=Round
  CAN2_SPTG_Sta : Outport
  wires:
  Data Type Conversion/1 -> CAN2_SPTG_Sta/1
  SPTGSta/1 -> Data Type Conversion/1

== system halout/HAL_OUT/CAN2/FD_BCM1_0x216/APMDoorControlSta ==
  APMDoorControlSta : Inport
  Data Type Conversion : DataTypeConversion  OutDataTypeStr=uint8  RndMeth=Round
  CAN2_APMDoorControlSta : Outport
  wires:
  Data Type Conversion/1 -> CAN2_APMDoorControlSta/1
  APMDoorControlSta/1 -> Data Type Conversion/1

== system halout/HAL_OUT/CAN2/FD_BCM1_0x216/AllDoorSW ==
  AllDoorSW : Inport
  Data Type Conversion : DataTypeConversion  OutDataTypeStr=uint8  RndMeth=Round
  CAN2_AllDoorSW : Outport
  wires:
  Data Type Conversion/1 -> CAN2_AllDoorSW/1
  AllDoorSW/1 -> Data Type Conversion/1

== system halout/HAL_OUT/CAN2/FD_BCM1_0x216/AntiTheftSeatFold ==
  AntiTheftSeatFold : Inport
  Data Type Conversion : DataTypeConversion  OutDataTypeStr=uint8  RndMeth=Round
  CAN2_AntiTheftSeatFold : Outport
  wires:
  Data Type Conversion/1 -> CAN2_AntiTheftSeatFold/1
  AntiTheftSeatFold/1 -> Data Type Conversion/1

== system halout/HAL_OUT/CAN2/FD_BCM1_0x216/AntitheftSta ==
  AntitheftSta : Inport
  Data Type Conversion : DataTypeConversion  OutDataTypeStr=uint8  RndMeth=Round
  CAN2_AntitheftSta : Outport
  wires:
  Data Type Conversion/1 -> CAN2_AntitheftSta/1
  AntitheftSta/1 -> Data Type Conversion/1

== system halout/HAL_OUT/CAN2/FD_BCM1_0x216/BCMBuzzerReq ==
  BCMBuzzerReq : Inport
  Data Type Conversion : DataTypeConversion  OutDataTypeStr=uint8  RndMeth=Round
  CAN2_BCM_Buzzer_Req : Outport
  wires:
  Data Type Conversion/1 -> CAN2_BCM_Buzzer_Req/1
  BCMBuzzerReq/1 -> Data Type Conversion/1

== system halout/HAL_OUT/CAN2/FD_BCM1_0x216/BCMDoorLockSta ==
  BCMDoorLockSta : Inport
  Data Type Conversion : DataTypeConversion  OutDataTypeStr=uint8  RndMeth=Round
  CAN2_BCM_DoorLock_Sta : Outport
  wires:
  Data Type Conversion/1 -> CAN2_BCM_DoorLock_Sta/1
  BCMDoorLockSta/1 -> Data Type Conversion/1

== system halout/HAL_OUT/CAN2/FD_BCM1_0x216/BrakeLamp ==
  BrakeLamp : Inport
  Data Type Conversion : DataTypeConversion  OutDataTypeStr=uint8  RndMeth=Round
  CAN2_BrakeLamp : Outport
  wires:
  Data Type Conversion/1 -> CAN2_BrakeLamp/1
  BrakeLamp/1 -> Data Type Conversion/1

== system halout/HAL_OUT/CAN2/FD_BCM1_0x216/CTDCtrl ==
  CTDCtrl : Inport
  Data Type Conversion : DataTypeConversion  OutDataTypeStr=uint8  RndMeth=Round
  CAN2_CTDCtrl : Outport
  wires:
  Data Type Conversion/1 -> CAN2_CTDCtrl/1
  CTDCtrl/1 -> Data Type Conversion/1

== system halout/HAL_OUT/CAN2/FD_BCM1_0x216/CTDLockSW ==
  CTDLockSW : Inport
  Data Type Conversion : DataTypeConversion  OutDataTypeStr=uint8  RndMeth=Round
  CAN2_CTDLockSW : Outport
  wires:
  Data Type Conversion/1 -> CAN2_CTDLockSW/1
  CTDLockSW/1 -> Data Type Conversion/1

== system halout/HAL_OUT/CAN2/FD_BCM1_0x216/CTDUnlockSW ==
  CTDUnlockSW : Inport
  Data Type Conversion : DataTypeConversion  OutDataTypeStr=uint8  RndMeth=Round
  CAN2_CTDUnlockSW : Outport
  wires:
  Data Type Conversion/1 -> CAN2_CTDUnlockSW/1
  CTDUnlockSW/1 -> Data Type Conversion/1

== system halout/HAL_OUT/CAN2/FD_BCM1_0x216/CrashDetd ==
  CrashDetd : Inport
  Data Type Conversion : DataTypeConversion  OutDataTypeStr=uint8  RndMeth=Round
  CAN2_CrashDetd : Outport
  wires:
  Data Type Conversion/1 -> CAN2_CrashDetd/1
  CrashDetd/1 -> Data Type Conversion/1

== system halout/HAL_OUT/CAN2/FD_BCM1_0x216/Dimmer ==
  Dimmer : Inport
  Data Type Conversion : DataTypeConversion  OutDataTypeStr=uint8  RndMeth=Round
  CAN2_Dimmer : Outport
  wires:
  Data Type Conversion/1 -> CAN2_Dimmer/1
  Dimmer/1 -> Data Type Conversion/1

== system halout/HAL_OUT/CAN2/FD_BCM1_0x216/DimmerEN ==
  DimmerEN : Inport
  Data Type Conversion : DataTypeConversion  OutDataTypeStr=uint8  RndMeth=Round
  CAN2_DimmerEN : Outport
  wires:
  Data Type Conversion/1 -> CAN2_DimmerEN/1
  DimmerEN/1 -> Data Type Conversion/1

== system halout/HAL_OUT/CAN2/FD_BCM1_0x216/DoorLockIND ==
  DoorLockIND : Inport
  Data Type Conversion : DataTypeConversion  OutDataTypeStr=uint8  RndMeth=Round
  CAN2_DoorLockIND : Outport
  wires:
  Data Type Conversion/1 -> CAN2_DoorLockIND/1
  DoorLockIND/1 -> Data Type Conversion/1

== system halout/HAL_OUT/CAN2/FD_BCM1_0x216/DrDoorSW ==
  DrDoorSW : Inport
  Data Type Conversion : DataTypeConversion  OutDataTypeStr=uint8  RndMeth=Round
  CAN2_DrDoorSW : Outport
  wires:
  Data Type Conversion/1 -> CAN2_DrDoorSW/1
  DrDoorSW/1 -> Data Type Conversion/1

== system halout/HAL_OUT/CAN2/FD_BCM1_0x216/FDCBCMLockAlarmCmd ==
  FDCBCMLockAlarmCmd : Inport
  Data Type Conversion : DataTypeConversion  OutDataTypeStr=uint8  RndMeth=Round
  CAN2_FDC_BCM_LockAlarm_Cmd : Outport
  wires:
  Data Type Conversion/1 -> CAN2_FDC_BCM_LockAlarm_Cmd/1
  FDCBCMLockAlarmCmd/1 -> Data Type Conversion/1

== system halout/HAL_OUT/CAN2/FD_BCM1_0x216/FDCTHCMAPTCWarningSta ==
  FDCTHCMAPTCWarningSta : Inport
  Data Type Conversion : DataTypeConversion  OutDataTypeStr=uint8  RndMeth=Round
  CAN2_FDC_THCM_APTCWarning_Sta : Outport
  wires:
  Data Type Conversion/1 -> CAN2_FDC_THCM_APTCWarning_Sta/1
  FDCTHCMAPTCWarningSta/1 -> Data Type Conversion/1

== system halout/HAL_OUT/CAN2/FD_BCM1_0x216/FollowMe ==
  FollowMe : Inport
  Data Type Conversion : DataTypeConversion  OutDataTypeStr=uint8  RndMeth=Round
  CAN2_FollowMe : Outport
  wires:
  Data Type Conversion/1 -> CAN2_FollowMe/1
  FollowMe/1 -> Data Type Conversion/1

== system halout/HAL_OUT/CAN2/FD_BCM1_0x216/FrChargingDoorCtrl ==
  FrChargingDoorCtrl : Inport
  Data Type Conversion : DataTypeConversion  OutDataTypeStr=uint8  RndMeth=Round
  CAN2_Fr_ChargingDoorCtrl : Outport
  wires:
  Data Type Conversion/1 -> CAN2_Fr_ChargingDoorCtrl/1
  FrChargingDoorCtrl/1 -> Data Type Conversion/1

== system halout/HAL_OUT/CAN2/FD_BCM1_0x216/FrFogLamp ==
  FrFogLamp : Inport
  Data Type Conversion : DataTypeConversion  OutDataTypeStr=uint8  RndMeth=Round
  CAN2_Fr_FogLamp : Outport
  wires:
  Data Type Conversion/1 -> CAN2_Fr_FogLamp/1
  FrFogLamp/1 -> Data Type Conversion/1

== system halout/HAL_OUT/CAN2/FD_BCM1_0x216/FrWiperH ==
  FrWiperH : Inport
  Data Type Conversion : DataTypeConversion  OutDataTypeStr=uint8  RndMeth=Round
  CAN2_Fr_Wiper_H : Outport
  wires:
  Data Type Conversion/1 -> CAN2_Fr_Wiper_H/1
  FrWiperH/1 -> Data Type Conversion/1

== system halout/HAL_OUT/CAN2/FD_BCM1_0x216/FrWiperL ==
  FrWiperL : Inport
  Data Type Conversion : DataTypeConversion  OutDataTypeStr=uint8  RndMeth=Round
  CAN2_Fr_Wiper_L : Outport
  wires:
  Data Type Conversion/1 -> CAN2_Fr_Wiper_L/1
  FrWiperL/1 -> Data Type Conversion/1

== system halout/HAL_OUT/CAN2/FD_BCM1_0x216/HBeam ==
  HBeam : Inport
  Data Type Conversion : DataTypeConversion  OutDataTypeStr=uint8  RndMeth=Round
  CAN2_H_Beam : Outport
  wires:
  Data Type Conversion/1 -> CAN2_H_Beam/1
  HBeam/1 -> Data Type Conversion/1

== system halout/HAL_OUT/CAN2/FD_BCM1_0x216/HazardSW ==
  HazardSW : Inport
  Data Type Conversion : DataTypeConversion  OutDataTypeStr=uint8  RndMeth=Round
  CAN2_HazardSW : Outport
  wires:
  Data Type Conversion/1 -> CAN2_HazardSW/1
  HazardSW/1 -> Data Type Conversion/1

== system halout/HAL_OUT/CAN2/FD_BCM1_0x216/HoodSW ==
  HoodSW : Inport
  Data Type Conversion : DataTypeConversion  OutDataTypeStr=uint8  RndMeth=Round
  CAN2_HoodSW : Outport
  wires:
  Data Type Conversion/1 -> CAN2_HoodSW/1
  HoodSW/1 -> Data Type Conversion/1

== system halout/HAL_OUT/CAN2/FD_BCM1_0x216/HornCtrl ==
  HornCtrl : Inport
  Data Type Conversion : DataTypeConversion  OutDataTypeStr=uint8  RndMeth=Round
  CAN2_HornCtrl : Outport
  wires:
  Data Type Conversion/1 -> CAN2_HornCtrl/1
  HornCtrl/1 -> Data Type Conversion/1

== system halout/HAL_OUT/CAN2/FD_BCM1_0x216/LAPMWdwEnable ==
  LAPMWdwEnable : Inport
  Data Type Conversion : DataTypeConversion  OutDataTypeStr=uint8  RndMeth=Round
  CAN2_L_APM_WdwEnable : Outport
  wires:
  Data Type Conversion/1 -> CAN2_L_APM_WdwEnable/1
  LAPMWdwEnable/1 -> Data Type Conversion/1

== system halout/HAL_OUT/CAN2/FD_BCM1_0x216/LBSD ==
  LBSD : Inport
  Data Type Conversion : DataTypeConversion  OutDataTypeStr=uint8  RndMeth=Round
  CAN2_LBSD : Outport
  wires:
  Data Type Conversion/1 -> CAN2_LBSD/1
  LBSD/1 -> Data Type Conversion/1

== system halout/HAL_OUT/CAN2/FD_BCM1_0x216/LBeam ==
  LBeam : Inport
  Data Type Conversion : DataTypeConversion  OutDataTypeStr=uint8  RndMeth=Round
  CAN2_L_Beam : Outport
  wires:
  Data Type Conversion/1 -> CAN2_L_Beam/1
  LBeam/1 -> Data Type Conversion/1

== system halout/HAL_OUT/CAN2/FD_BCM1_0x216/LDRL ==
  LDRL : Inport
  Data Type Conversion : DataTypeConversion  OutDataTypeStr=uint8  RndMeth=Round
  CAN2_LDRL : Outport
  wires:
  Data Type Conversion/1 -> CAN2_LDRL/1
  LDRL/1 -> Data Type Conversion/1

== system halout/HAL_OUT/CAN2/FD_BCM1_0x216/LTurnLP ==
  LTurnLP : Inport
  Data Type Conversion : DataTypeConversion  OutDataTypeStr=uint8  RndMeth=Round
  CAN2_LTurnLP : Outport
  wires:
  Data Type Conversion/1 -> CAN2_LTurnLP/1
  LTurnLP/1 -> Data Type Conversion/1

== system halout/HAL_OUT/CAN2/FD_BCM1_0x216/LockSetting ==
  LockSetting : Inport
  Data Type Conversion : DataTypeConversion  OutDataTypeStr=uint8  RndMeth=Round
  CAN2_LockSetting : Outport
  wires:
  Data Type Conversion/1 -> CAN2_LockSetting/1
  LockSetting/1 -> Data Type Conversion/1

== system halout/HAL_OUT/CAN2/FD_BCM1_0x216/MirrorCtrl ==
  MirrorCtrl : Inport
  Data Type Conversion : DataTypeConversion  OutDataTypeStr=uint8  RndMeth=Round
  CAN2_MirrorCtrl : Outport
  wires:
  Data Type Conversion/1 -> CAN2_MirrorCtrl/1
  MirrorCtrl/1 -> Data Type Conversion/1

== system halout/HAL_OUT/CAN2/FD_BCM1_0x216/MirrorDefog ==
  MirrorDefog : Inport
  Data Type Conversion : DataTypeConversion  OutDataTypeStr=uint8  RndMeth=Round
  CAN2_MirrorDefog : Outport
  wires:
  Data Type Conversion/1 -> CAN2_MirrorDefog/1
  MirrorDefog/1 -> Data Type Conversion/1

== system halout/HAL_OUT/CAN2/FD_BCM1_0x216/PosLamp ==
  PosLamp : Inport
  Data Type Conversion : DataTypeConversion  OutDataTypeStr=uint8  RndMeth=Round
  CAN2_PosLamp : Outport
  wires:
  Data Type Conversion/1 -> CAN2_PosLamp/1
  PosLamp/1 -> Data Type Conversion/1

== system halout/HAL_OUT/CAN2/FD_BCM1_0x216/PsDoorSW ==
  PsDoorSW : Inport
  Data Type Conversion : DataTypeConversion  OutDataTypeStr=uint8  RndMeth=Round
  CAN2_PsDoorSW : Outport
  wires:
  Data Type Conversion/1 -> CAN2_PsDoorSW/1
  PsDoorSW/1 -> Data Type Conversion/1

== system halout/HAL_OUT/CAN2/FD_BCM1_0x216/RBSD ==
  RBSD : Inport
  Data Type Conversion : DataTypeConversion  OutDataTypeStr=uint8  RndMeth=Round
  CAN2_RBSD : Outport
  wires:
  Data Type Conversion/1 -> CAN2_RBSD/1
  RBSD/1 -> Data Type Conversion/1

== system halout/HAL_OUT/CAN2/FD_BCM1_0x216/RDRL ==
  RDRL : Inport
  Data Type Conversion : DataTypeConversion  OutDataTypeStr=uint8  RndMeth=Round
  CAN2_RDRL : Outport
  wires:
  Data Type Conversion/1 -> CAN2_RDRL/1
  RDRL/1 -> Data Type Conversion/1

== system halout/HAL_OUT/CAN2/FD_BCM1_0x216/RLDoorSW ==
  RLDoorSW : Inport
  Data Type Conversion : DataTypeConversion  OutDataTypeStr=uint8  RndMeth=Round
  CAN2_RLDoorSW : Outport
  wires:
  Data Type Conversion/1 -> CAN2_RLDoorSW/1
  RLDoorSW/1 -> Data Type Conversion/1

== system halout/HAL_OUT/CAN2/FD_BCM1_0x216/RRDoorSW ==
  RRDoorSW : Inport
  Data Type Conversion : DataTypeConversion  OutDataTypeStr=uint8  RndMeth=Round
  CAN2_RRDoorSW : Outport
  wires:
  Data Type Conversion/1 -> CAN2_RRDoorSW/1
  RRDoorSW/1 -> Data Type Conversion/1

== system halout/HAL_OUT/CAN2/FD_BCM1_0x216/RTurnLP ==
  RTurnLP : Inport
  Data Type Conversion : DataTypeConversion  OutDataTypeStr=uint8  RndMeth=Round
  CAN2_RTurnLP : Outport
  wires:
  Data Type Conversion/1 -> CAN2_RTurnLP/1
  RTurnLP/1 -> Data Type Conversion/1

== system halout/HAL_OUT/CAN2/FD_BCM1_0x216/ReverseLamp ==
  ReverseLamp : Inport
  Data Type Conversion : DataTypeConversion  OutDataTypeStr=uint8  RndMeth=Round
  CAN2_ReverseLamp : Outport
  wires:
  Data Type Conversion/1 -> CAN2_ReverseLamp/1
  ReverseLamp/1 -> Data Type Conversion/1

== system halout/HAL_OUT/CAN2/FD_BCM1_0x216/RoomLampH ==
  RoomLampH : Inport
  Data Type Conversion : DataTypeConversion  OutDataTypeStr=uint8  RndMeth=Round
  CAN2_RoomLampH : Outport
  wires:
  Data Type Conversion/1 -> CAN2_RoomLampH/1
  RoomLampH/1 -> Data Type Conversion/1

== system halout/HAL_OUT/CAN2/FD_BCM1_0x216/RoomLampL ==
  RoomLampL : Inport
  Data Type Conversion : DataTypeConversion  OutDataTypeStr=uint8  RndMeth=Round
  CAN2_RoomLampL : Outport
  wires:
  Data Type Conversion/1 -> CAN2_RoomLampL/1
  RoomLampL/1 -> Data Type Conversion/1

== system halout/HAL_OUT/CAN2/FD_BCM1_0x216/RrChargingDoorCtrl ==
  RrChargingDoorCtrl : Inport
  Data Type Conversion : DataTypeConversion  OutDataTypeStr=uint8  RndMeth=Round
  CAN2_Rr_ChargingDoorCtrl : Outport
  wires:
  Data Type Conversion/1 -> CAN2_Rr_ChargingDoorCtrl/1
  RrChargingDoorCtrl/1 -> Data Type Conversion/1

== system halout/HAL_OUT/CAN2/FD_BCM1_0x216/RrDefog ==
  RrDefog : Inport
  Data Type Conversion : DataTypeConversion  OutDataTypeStr=uint8  RndMeth=Round
  CAN2_Rr_Defog : Outport
  wires:
  Data Type Conversion/1 -> CAN2_Rr_Defog/1
  RrDefog/1 -> Data Type Conversion/1

== system halout/HAL_OUT/CAN2/FD_BCM1_0x216/RrFogLamp ==
  RrFogLamp : Inport
  Data Type Conversion : DataTypeConversion  OutDataTypeStr=uint8  RndMeth=Round
  CAN2_Rr_FogLamp : Outport
  wires:
  Data Type Conversion/1 -> CAN2_Rr_FogLamp/1
  RrFogLamp/1 -> Data Type Conversion/1

== system halout/HAL_OUT/CAN2/FD_BCM1_0x216/RrWiper ==
  RrWiper : Inport
  Data Type Conversion : DataTypeConversion  OutDataTypeStr=uint8  RndMeth=Round
  CAN2_Rr_Wiper : Outport
  wires:
  Data Type Conversion/1 -> CAN2_Rr_Wiper/1
  RrWiper/1 -> Data Type Conversion/1

== system halout/HAL_OUT/CAN2/FD_BCM1_0x216/TailgateHDSW ==
  TailgateHDSW : Inport
  Data Type Conversion : DataTypeConversion  OutDataTypeStr=uint8  RndMeth=Round
  CAN2_TailgateHDSW : Outport
  wires:
  Data Type Conversion/1 -> CAN2_TailgateHDSW/1
  TailgateHDSW/1 -> Data Type Conversion/1

== system halout/HAL_OUT/CAN2/FD_BCM1_0x216/TailgateRemote ==
  TailgateRemote : Inport
  Data Type Conversion : DataTypeConversion  OutDataTypeStr=uint8  RndMeth=Round
  CAN2_TailgateRemote : Outport
  wires:
  Data Type Conversion/1 -> CAN2_TailgateRemote/1
  TailgateRemote/1 -> Data Type Conversion/1

== system halout/HAL_OUT/CAN2/FD_BCM1_0x216/TailgateSW ==
  TailgateSW : Inport
  Data Type Conversion : DataTypeConversion  OutDataTypeStr=uint8  RndMeth=Round
  CAN2_Tailgate_SW : Outport
  wires:
  Data Type Conversion/1 -> CAN2_Tailgate_SW/1
  TailgateSW/1 -> Data Type Conversion/1

== system halout/HAL_OUT/CAN2/FD_BCM1_0x216/TrunkRel ==
  TrunkRel : Inport
  Data Type Conversion : DataTypeConversion  OutDataTypeStr=uint8  RndMeth=Round
  CAN2_TrunkRel : Outport
  wires:
  Data Type Conversion/1 -> CAN2_TrunkRel/1
  TrunkRel/1 -> Data Type Conversion/1

== system halout/HAL_OUT/CAN2/FD_BCM1_0x216/WasherCtrl ==
  WasherCtrl : Inport
  Data Type Conversion : DataTypeConversion  OutDataTypeStr=uint8  RndMeth=Round
  CAN2_WasherCtrl : Outport
  wires:
  Data Type Conversion/1 -> CAN2_WasherCtrl/1
  WasherCtrl/1 -> Data Type Conversion/1

== system halout/HAL_OUT/CAN2/FD_BCM1_0x216/WiperFixMode ==
  WiperFixMode : Inport
  Data Type Conversion : DataTypeConversion  OutDataTypeStr=uint8  RndMeth=Round
  CAN2_WiperFixMode : Outport
  wires:
  Data Type Conversion/1 -> CAN2_WiperFixMode/1
  WiperFixMode/1 -> Data Type Conversion/1

== system halout/HAL_OUT/CAN2/FD_BCM2_0x217/AmbLightBreath1 ==
  AmbLightBreath1 : Inport
  Data Type Conversion : DataTypeConversion  OutDataTypeStr=uint8  RndMeth=Round
  CAN2_AmbLightBreath1 : Outport
  wires:
  Data Type Conversion/1 -> CAN2_AmbLightBreath1/1
  AmbLightBreath1/1 -> Data Type Conversion/1
